simulink model "LIP"  (R2025b)
settings: Solver=FixedStepAuto  StartTime=0.0  StopTime=inf  FixedStep=1E-2  RelTol=1e-3
undefined symbols (not defined in the file or in its folder): Busy, Wait
libraries: aerolibanimutils x1
settings Model: Creator=abstract  LastModifiedBy=abstract

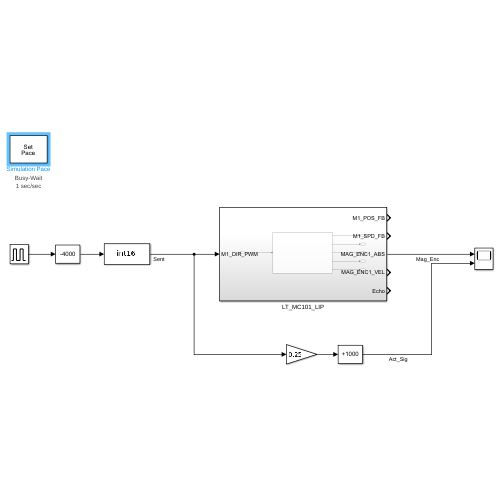
[thumbnail: Simulink's stored preview of the top-level diagram]
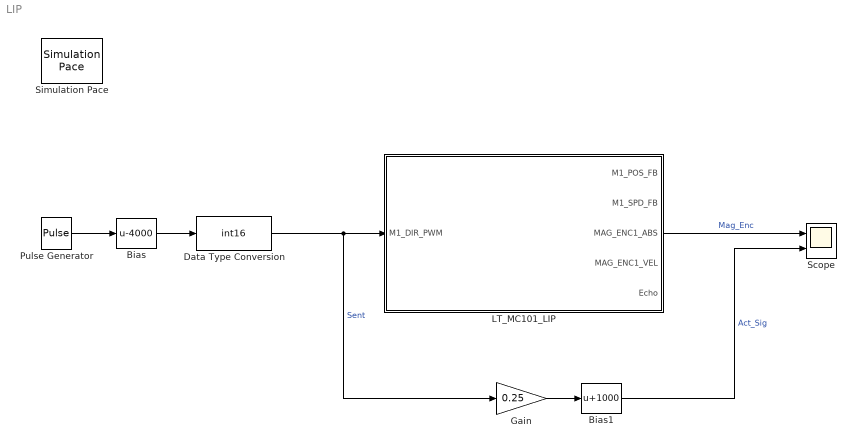
== system LIP ==
  Bias : Bias  Bias=-4000  SaturateOnIntegerOverflow=off
  Bias1 : Bias  Bias=1000  SaturateOnIntegerOverflow=off
  Data Type Conversion : DataTypeConversion  OutDataTypeStr=int16  SaturateOnIntegerOverflow=off  RndMeth=Floor
  Gain : Gain  Gain=0.25
  LT_MC101_LIP : Subsystem
  Pulse Generator : DiscretePulseGenerator  PulseType=Time based  Amplitude=8000  Period=1  PulseWidth=50
  Scope : Scope  NumInputPorts=2
      settings: ActiveDisplayYMinimum=1719.9898028254006  ActiveDisplayYMaximum=2092.7594493001875
  Simulation Pace : aerolibanimutils/Simulation Pace  SimulationPace=1  SleepMode=Busy-Wait  OutputPaceError=off  SampleTime=-1
  wires:
  Pulse Generator/1 -> Bias/1
  Data Type Conversion/1 -> LT_MC101_LIP/1(M1_DIR_PWM), Gain/1  "Sent"
  Bias/1 -> Data Type Conversion/1
  LT_MC101_LIP/3(MAG_ENC1_ABS) -> Scope/1  "Mag_Enc"
  Gain/1 -> Bias1/1
  Bias1/1 -> Scope/2  "Act_Sig"

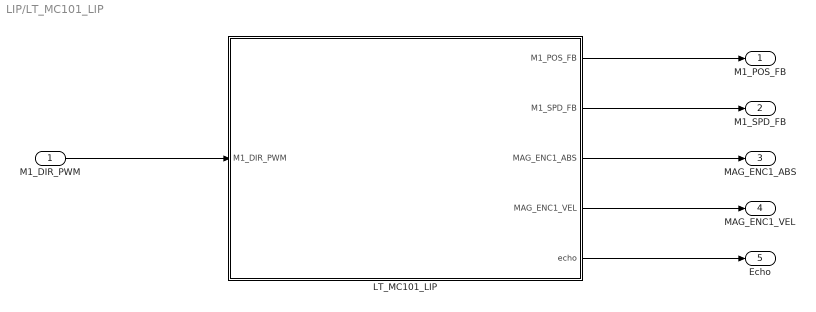
== system LIP/LT_MC101_LIP ==
  M1_DIR_PWM : Inport  OutDataTypeStr=int16
  LT_MC101_LIP : MATLAB Function  TreatAsAtomicUnit=on
  M1_POS_FB : Outport  OutDataTypeStr=int32
  M1_SPD_FB : Outport  Port=2  OutDataTypeStr=int32
  MAG_ENC1_ABS : Outport  Port=3  OutDataTypeStr=uint16
  MAG_ENC1_VEL : Outport  Port=4  OutDataTypeStr=single
  Echo : Outport  Port=5  OutDataTypeStr=single
  wires:
  M1_DIR_PWM/1 -> LT_MC101_LIP/1(M1_DIR_PWM)
  LT_MC101_LIP/1(M1_POS_FB) -> M1_POS_FB/1
  LT_MC101_LIP/2(M1_SPD_FB) -> M1_SPD_FB/1
  LT_MC101_LIP/3(MAG_ENC1_ABS) -> MAG_ENC1_ABS/1
  LT_MC101_LIP/4(MAG_ENC1_VEL) -> MAG_ENC1_VEL/1
  LT_MC101_LIP/5(echo) -> Echo/1

== matlab function LIP/LT_MC101_LIP/LT_MC101_LIP ==
  data: M1_DIR_PWM input; M1_POS_FB output; M1_SPD_FB output; MAG_ENC1_ABS output; MAG_ENC1_VEL output; echo output
function [M1_POS_FB, M1_SPD_FB, MAG_ENC1_ABS, MAG_ENC1_VEL, echo] = LT_MC101_LIP(M1_DIR_PWM)

arguments (Input)
    M1_DIR_PWM (1, 1) int16
end

Set_LIP_M1(M1_DIR_PWM);
% Set_LIP_Echo(single(M1_DIR_PWM));

[M1_POS_FB, M1_SPD_FB, MAG_ENC1_ABS, MAG_ENC1_VEL, echo] = Get_LIP_State();
